simulink subsystem "LQR"  (R2024a)
settings: Solver=VariableStepAuto  StartTime=0.0  StopTime=10.0  RelTol=1e-3
undefined symbols (not defined in the file or in its folder): K_lqr
settings Model: Creator=Peter  LastModifiedBy=Peter

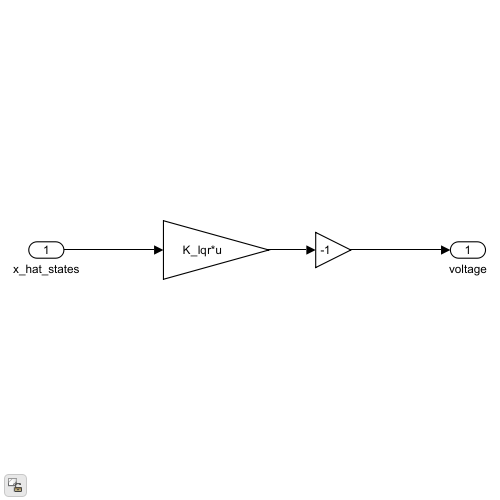
[thumbnail: Simulink's stored preview of the top-level diagram]
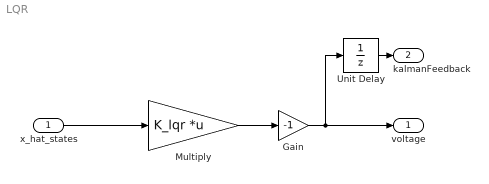
== system LQR ==
  x_hat_states : Inport
  Gain : Gain  Gain=-1
  Multiply : Gain  Gain=K_lqr  Multiplication=Matrix(K*u)
  Unit Delay : UnitDelay  SampleTime=-1  HasFrameUpgradeWarning=on
  voltage : Outport
  kalmanFeedback : Outport  Port=2  OutDataTypeStr=single
  wires:
  x_hat_states/1 -> Multiply/1
  Multiply/1 -> Gain/1
  Gain/1 -> voltage/1, Unit Delay/1
  Unit Delay/1 -> kalmanFeedback/1
